simulink model "ssc_battery_rom_qbat"  (R2021a)
settings: Solver=ode1be  StartTime=0.0  StopTime=3600  FixedStep=elec_dt  RelTol=1e-3
PreLoadFcn:
  | % Model parameters
  | ssc_battery_rom_qbat_param
undefined symbols (not defined in the file or in its folder): coolant_flow_qoff, coolant_flow_Toff, coolant_flow_Ton, elec_dt, heat_dt, iniBatteryTemp, iniCoolantTemp, R0_mat, sigbuilder_block, SOC_vec, T_vec, V0_mat
libraries: fl_lib x47, nesl_utility x47, ee_lib x14
(part 3 of 3)

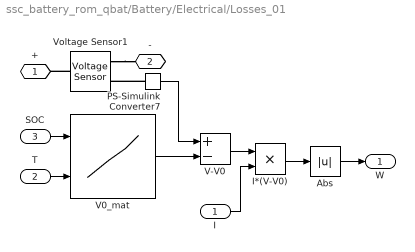
== system ssc_battery_rom_qbat/Battery/Electrical/Losses_01 ==
  I : Inport
  T : Inport  Port=2
  SOC : Inport  Port=3
  Abs : Abs
  I*(V-V0) : Product
  PS-Simulink Converter7 : nesl_utility/PS-Simulink Converter  PhysicalDomain=network_engine_domain  SubClassName=ps_output  LeftPortType=input  RightPortType=output  PseudoPeriodic=off  Frequencies=[]  Unit=inherit  AffineConversion=off
      settings: SourceProductBaseCode=PW,SS
  V-V0 : Sum  Inputs=+-
  V0_mat : Lookup_n-D  BreakpointsForDimension1=SOC_vec  BreakpointsForDimension2=T_vec  Table=V0_mat  InternalRulePriority=Speed  RndMeth=Simplest  InputSameDT=on
      settings: InputPortMap=u0,u1
  Voltage Sensor1 : fl_lib/Electrical/Electrical Sensors/Voltage Sensor
  + : PMIOPort  Side=Left
  - : PMIOPort  Port=2  Side=Right
  W : Outport
  wires:
  Abs/1 -> W/1
  PS-Simulink Converter7/1 -> V-V0/1
  I/1 -> I*(V-V0)/2
  I*(V-V0)/1 -> Abs/1
  V-V0/1 -> I*(V-V0)/1
  V0_mat/1 -> V-V0/2
  SOC/1 -> V0_mat/1
  T/1 -> V0_mat/2
  connections:
  PS-Simulink Converter7/LConn1 -- Voltage Sensor1/RConn1
  Voltage Sensor1/RConn2 -- -/RConn1
  Voltage Sensor1/LConn1 -- +/RConn1

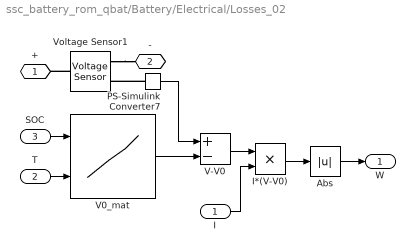
== system ssc_battery_rom_qbat/Battery/Electrical/Losses_02 ==
  I : Inport
  T : Inport  Port=2
  SOC : Inport  Port=3
  Abs : Abs
  I*(V-V0) : Product
  PS-Simulink Converter7 : nesl_utility/PS-Simulink Converter  PhysicalDomain=network_engine_domain  SubClassName=ps_output  LeftPortType=input  RightPortType=output  PseudoPeriodic=off  Frequencies=[]  Unit=inherit  AffineConversion=off
      settings: SourceProductBaseCode=PW,SS
  V-V0 : Sum  Inputs=+-
  V0_mat : Lookup_n-D  BreakpointsForDimension1=SOC_vec  BreakpointsForDimension2=T_vec  Table=V0_mat  InternalRulePriority=Speed  RndMeth=Simplest  InputSameDT=on
      settings: InputPortMap=u0,u1
  Voltage Sensor1 : fl_lib/Electrical/Electrical Sensors/Voltage Sensor
  + : PMIOPort  Side=Left
  - : PMIOPort  Port=2  Side=Right
  W : Outport
  wires:
  Abs/1 -> W/1
  PS-Simulink Converter7/1 -> V-V0/1
  I/1 -> I*(V-V0)/2
  I*(V-V0)/1 -> Abs/1
  V-V0/1 -> I*(V-V0)/1
  V0_mat/1 -> V-V0/2
  SOC/1 -> V0_mat/1
  T/1 -> V0_mat/2
  connections:
  PS-Simulink Converter7/LConn1 -- Voltage Sensor1/RConn1
  Voltage Sensor1/RConn2 -- -/RConn1
  Voltage Sensor1/LConn1 -- +/RConn1

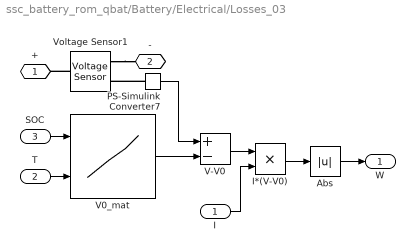
== system ssc_battery_rom_qbat/Battery/Electrical/Losses_03 ==
  I : Inport
  T : Inport  Port=2
  SOC : Inport  Port=3
  Abs : Abs
  I*(V-V0) : Product
  PS-Simulink Converter7 : nesl_utility/PS-Simulink Converter  PhysicalDomain=network_engine_domain  SubClassName=ps_output  LeftPortType=input  RightPortType=output  PseudoPeriodic=off  Frequencies=[]  Unit=inherit  AffineConversion=off
      settings: SourceProductBaseCode=PW,SS
  V-V0 : Sum  Inputs=+-
  V0_mat : Lookup_n-D  BreakpointsForDimension1=SOC_vec  BreakpointsForDimension2=T_vec  Table=V0_mat  InternalRulePriority=Speed  RndMeth=Simplest  InputSameDT=on
      settings: InputPortMap=u0,u1
  Voltage Sensor1 : fl_lib/Electrical/Electrical Sensors/Voltage Sensor
  + : PMIOPort  Side=Left
  - : PMIOPort  Port=2  Side=Right
  W : Outport
  wires:
  Abs/1 -> W/1
  PS-Simulink Converter7/1 -> V-V0/1
  I/1 -> I*(V-V0)/2
  I*(V-V0)/1 -> Abs/1
  V-V0/1 -> I*(V-V0)/1
  V0_mat/1 -> V-V0/2
  SOC/1 -> V0_mat/1
  T/1 -> V0_mat/2
  connections:
  PS-Simulink Converter7/LConn1 -- Voltage Sensor1/RConn1
  Voltage Sensor1/RConn2 -- -/RConn1
  Voltage Sensor1/LConn1 -- +/RConn1

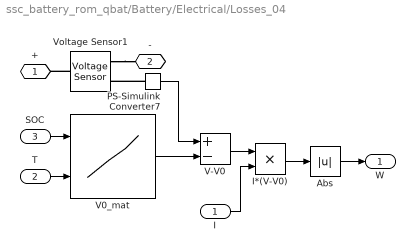
== system ssc_battery_rom_qbat/Battery/Electrical/Losses_04 ==
  I : Inport
  T : Inport  Port=2
  SOC : Inport  Port=3
  Abs : Abs
  I*(V-V0) : Product
  PS-Simulink Converter7 : nesl_utility/PS-Simulink Converter  PhysicalDomain=network_engine_domain  SubClassName=ps_output  LeftPortType=input  RightPortType=output  PseudoPeriodic=off  Frequencies=[]  Unit=inherit  AffineConversion=off
      settings: SourceProductBaseCode=PW,SS
  V-V0 : Sum  Inputs=+-
  V0_mat : Lookup_n-D  BreakpointsForDimension1=SOC_vec  BreakpointsForDimension2=T_vec  Table=V0_mat  InternalRulePriority=Speed  RndMeth=Simplest  InputSameDT=on
      settings: InputPortMap=u0,u1
  Voltage Sensor1 : fl_lib/Electrical/Electrical Sensors/Voltage Sensor
  + : PMIOPort  Side=Left
  - : PMIOPort  Port=2  Side=Right
  W : Outport
  wires:
  Abs/1 -> W/1
  PS-Simulink Converter7/1 -> V-V0/1
  I/1 -> I*(V-V0)/2
  I*(V-V0)/1 -> Abs/1
  V-V0/1 -> I*(V-V0)/1
  V0_mat/1 -> V-V0/2
  SOC/1 -> V0_mat/1
  T/1 -> V0_mat/2
  connections:
  PS-Simulink Converter7/LConn1 -- Voltage Sensor1/RConn1
  Voltage Sensor1/RConn2 -- -/RConn1
  Voltage Sensor1/LConn1 -- +/RConn1

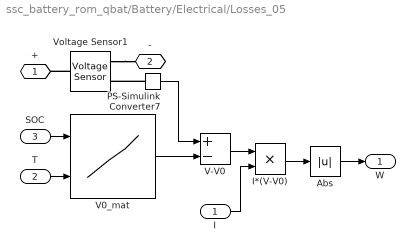
== system ssc_battery_rom_qbat/Battery/Electrical/Losses_05 ==
  I : Inport
  T : Inport  Port=2
  SOC : Inport  Port=3
  Abs : Abs
  I*(V-V0) : Product
  PS-Simulink Converter7 : nesl_utility/PS-Simulink Converter  PhysicalDomain=network_engine_domain  SubClassName=ps_output  LeftPortType=input  RightPortType=output  PseudoPeriodic=off  Frequencies=[]  Unit=inherit  AffineConversion=off
      settings: SourceProductBaseCode=PW,SS
  V-V0 : Sum  Inputs=+-
  V0_mat : Lookup_n-D  BreakpointsForDimension1=SOC_vec  BreakpointsForDimension2=T_vec  Table=V0_mat  InternalRulePriority=Speed  RndMeth=Simplest  InputSameDT=on
      settings: InputPortMap=u0,u1
  Voltage Sensor1 : fl_lib/Electrical/Electrical Sensors/Voltage Sensor
  + : PMIOPort  Side=Left
  - : PMIOPort  Port=2  Side=Right
  W : Outport
  wires:
  Abs/1 -> W/1
  PS-Simulink Converter7/1 -> V-V0/1
  I/1 -> I*(V-V0)/2
  I*(V-V0)/1 -> Abs/1
  V-V0/1 -> I*(V-V0)/1
  V0_mat/1 -> V-V0/2
  SOC/1 -> V0_mat/1
  T/1 -> V0_mat/2
  connections:
  PS-Simulink Converter7/LConn1 -- Voltage Sensor1/RConn1
  Voltage Sensor1/RConn2 -- -/RConn1
  Voltage Sensor1/LConn1 -- +/RConn1

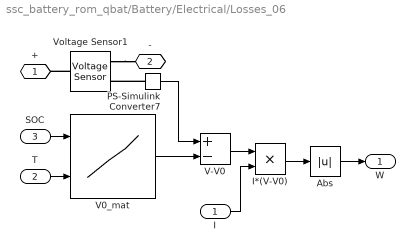
== system ssc_battery_rom_qbat/Battery/Electrical/Losses_06 ==
  I : Inport
  T : Inport  Port=2
  SOC : Inport  Port=3
  Abs : Abs
  I*(V-V0) : Product
  PS-Simulink Converter7 : nesl_utility/PS-Simulink Converter  PhysicalDomain=network_engine_domain  SubClassName=ps_output  LeftPortType=input  RightPortType=output  PseudoPeriodic=off  Frequencies=[]  Unit=inherit  AffineConversion=off
      settings: SourceProductBaseCode=PW,SS
  V-V0 : Sum  Inputs=+-
  V0_mat : Lookup_n-D  BreakpointsForDimension1=SOC_vec  BreakpointsForDimension2=T_vec  Table=V0_mat  InternalRulePriority=Speed  RndMeth=Simplest  InputSameDT=on
      settings: InputPortMap=u0,u1
  Voltage Sensor1 : fl_lib/Electrical/Electrical Sensors/Voltage Sensor
  + : PMIOPort  Side=Left
  - : PMIOPort  Port=2  Side=Right
  W : Outport
  wires:
  Abs/1 -> W/1
  PS-Simulink Converter7/1 -> V-V0/1
  I/1 -> I*(V-V0)/2
  I*(V-V0)/1 -> Abs/1
  V-V0/1 -> I*(V-V0)/1
  V0_mat/1 -> V-V0/2
  SOC/1 -> V0_mat/1
  T/1 -> V0_mat/2
  connections:
  PS-Simulink Converter7/LConn1 -- Voltage Sensor1/RConn1
  Voltage Sensor1/RConn2 -- -/RConn1
  Voltage Sensor1/LConn1 -- +/RConn1

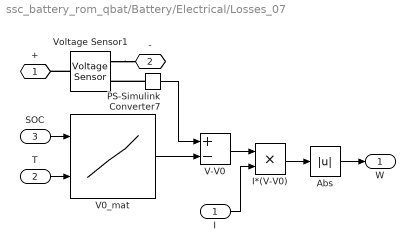
== system ssc_battery_rom_qbat/Battery/Electrical/Losses_07 ==
  I : Inport
  T : Inport  Port=2
  SOC : Inport  Port=3
  Abs : Abs
  I*(V-V0) : Product
  PS-Simulink Converter7 : nesl_utility/PS-Simulink Converter  PhysicalDomain=network_engine_domain  SubClassName=ps_output  LeftPortType=input  RightPortType=output  PseudoPeriodic=off  Frequencies=[]  Unit=inherit  AffineConversion=off
      settings: SourceProductBaseCode=PW,SS
  V-V0 : Sum  Inputs=+-
  V0_mat : Lookup_n-D  BreakpointsForDimension1=SOC_vec  BreakpointsForDimension2=T_vec  Table=V0_mat  InternalRulePriority=Speed  RndMeth=Simplest  InputSameDT=on
      settings: InputPortMap=u0,u1
  Voltage Sensor1 : fl_lib/Electrical/Electrical Sensors/Voltage Sensor
  + : PMIOPort  Side=Left
  - : PMIOPort  Port=2  Side=Right
  W : Outport
  wires:
  Abs/1 -> W/1
  PS-Simulink Converter7/1 -> V-V0/1
  I/1 -> I*(V-V0)/2
  I*(V-V0)/1 -> Abs/1
  V-V0/1 -> I*(V-V0)/1
  V0_mat/1 -> V-V0/2
  SOC/1 -> V0_mat/1
  T/1 -> V0_mat/2
  connections:
  PS-Simulink Converter7/LConn1 -- Voltage Sensor1/RConn1
  Voltage Sensor1/RConn2 -- -/RConn1
  Voltage Sensor1/LConn1 -- +/RConn1

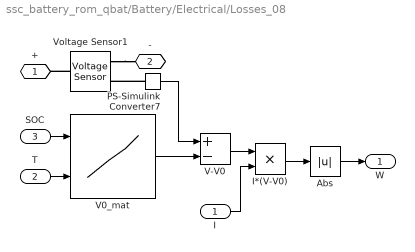
== system ssc_battery_rom_qbat/Battery/Electrical/Losses_08 ==
  I : Inport
  T : Inport  Port=2
  SOC : Inport  Port=3
  Abs : Abs
  I*(V-V0) : Product
  PS-Simulink Converter7 : nesl_utility/PS-Simulink Converter  PhysicalDomain=network_engine_domain  SubClassName=ps_output  LeftPortType=input  RightPortType=output  PseudoPeriodic=off  Frequencies=[]  Unit=inherit  AffineConversion=off
      settings: SourceProductBaseCode=PW,SS
  V-V0 : Sum  Inputs=+-
  V0_mat : Lookup_n-D  BreakpointsForDimension1=SOC_vec  BreakpointsForDimension2=T_vec  Table=V0_mat  InternalRulePriority=Speed  RndMeth=Simplest  InputSameDT=on
      settings: InputPortMap=u0,u1
  Voltage Sensor1 : fl_lib/Electrical/Electrical Sensors/Voltage Sensor
  + : PMIOPort  Side=Left
  - : PMIOPort  Port=2  Side=Right
  W : Outport
  wires:
  Abs/1 -> W/1
  PS-Simulink Converter7/1 -> V-V0/1
  I/1 -> I*(V-V0)/2
  I*(V-V0)/1 -> Abs/1
  V-V0/1 -> I*(V-V0)/1
  V0_mat/1 -> V-V0/2
  SOC/1 -> V0_mat/1
  T/1 -> V0_mat/2
  connections:
  PS-Simulink Converter7/LConn1 -- Voltage Sensor1/RConn1
  Voltage Sensor1/RConn2 -- -/RConn1
  Voltage Sensor1/LConn1 -- +/RConn1

== system ssc_battery_rom_qbat/Battery/Electrical/Losses_09 ==
  I : Inport
  T : Inport  Port=2
  SOC : Inport  Port=3
  Abs : Abs
  I*(V-V0) : Product
  PS-Simulink Converter7 : nesl_utility/PS-Simulink Converter  PhysicalDomain=network_engine_domain  SubClassName=ps_output  LeftPortType=input  RightPortType=output  PseudoPeriodic=off  Frequencies=[]  Unit=inherit  AffineConversion=off
      settings: SourceProductBaseCode=PW,SS
  V-V0 : Sum  Inputs=+-
  V0_mat : Lookup_n-D  BreakpointsForDimension1=SOC_vec  BreakpointsForDimension2=T_vec  Table=V0_mat  InternalRulePriority=Speed  RndMeth=Simplest  InputSameDT=on
      settings: InputPortMap=u0,u1
  Voltage Sensor1 : fl_lib/Electrical/Electrical Sensors/Voltage Sensor
  + : PMIOPort  Side=Left
  - : PMIOPort  Port=2  Side=Right
  W : Outport
  wires:
  Abs/1 -> W/1
  PS-Simulink Converter7/1 -> V-V0/1
  I/1 -> I*(V-V0)/2
  I*(V-V0)/1 -> Abs/1
  V-V0/1 -> I*(V-V0)/1
  V0_mat/1 -> V-V0/2
  SOC/1 -> V0_mat/1
  T/1 -> V0_mat/2
  connections:
  PS-Simulink Converter7/LConn1 -- Voltage Sensor1/RConn1
  Voltage Sensor1/RConn2 -- -/RConn1
  Voltage Sensor1/LConn1 -- +/RConn1

== system ssc_battery_rom_qbat/Battery/Electrical/Losses_10 ==
  I : Inport
  T : Inport  Port=2
  SOC : Inport  Port=3
  Abs : Abs
  I*(V-V0) : Product
  PS-Simulink Converter7 : nesl_utility/PS-Simulink Converter  PhysicalDomain=network_engine_domain  SubClassName=ps_output  LeftPortType=input  RightPortType=output  PseudoPeriodic=off  Frequencies=[]  Unit=inherit  AffineConversion=off
      settings: SourceProductBaseCode=PW,SS
  V-V0 : Sum  Inputs=+-
  V0_mat : Lookup_n-D  BreakpointsForDimension1=SOC_vec  BreakpointsForDimension2=T_vec  Table=V0_mat  InternalRulePriority=Speed  RndMeth=Simplest  InputSameDT=on
      settings: InputPortMap=u0,u1
  Voltage Sensor1 : fl_lib/Electrical/Electrical Sensors/Voltage Sensor
  + : PMIOPort  Side=Left
  - : PMIOPort  Port=2  Side=Right
  W : Outport
  wires:
  PS-Simulink Converter7/1 -> V-V0/1
  I/1 -> I*(V-V0)/2
  I*(V-V0)/1 -> Abs/1
  V-V0/1 -> I*(V-V0)/1
  V0_mat/1 -> V-V0/2
  SOC/1 -> V0_mat/1
  T/1 -> V0_mat/2
  Abs/1 -> W/1
  connections:
  PS-Simulink Converter7/LConn1 -- Voltage Sensor1/RConn1
  Voltage Sensor1/RConn2 -- -/RConn1
  Voltage Sensor1/LConn1 -- +/RConn1

== system ssc_battery_rom_qbat/Battery/Electrical/Losses_11 ==
  I : Inport
  T : Inport  Port=2
  SOC : Inport  Port=3
  Abs : Abs
  I*(V-V0) : Product
  PS-Simulink Converter7 : nesl_utility/PS-Simulink Converter  PhysicalDomain=network_engine_domain  SubClassName=ps_output  LeftPortType=input  RightPortType=output  PseudoPeriodic=off  Frequencies=[]  Unit=inherit  AffineConversion=off
      settings: SourceProductBaseCode=PW,SS
  V-V0 : Sum  Inputs=+-
  V0_mat : Lookup_n-D  BreakpointsForDimension1=SOC_vec  BreakpointsForDimension2=T_vec  Table=V0_mat  InternalRulePriority=Speed  RndMeth=Simplest  InputSameDT=on
      settings: InputPortMap=u0,u1
  Voltage Sensor1 : fl_lib/Electrical/Electrical Sensors/Voltage Sensor
  + : PMIOPort  Side=Left
  - : PMIOPort  Port=2  Side=Right
  W : Outport
  wires:
  Abs/1 -> W/1
  PS-Simulink Converter7/1 -> V-V0/1
  I/1 -> I*(V-V0)/2
  I*(V-V0)/1 -> Abs/1
  V-V0/1 -> I*(V-V0)/1
  V0_mat/1 -> V-V0/2
  SOC/1 -> V0_mat/1
  T/1 -> V0_mat/2
  connections:
  PS-Simulink Converter7/LConn1 -- Voltage Sensor1/RConn1
  Voltage Sensor1/RConn2 -- -/RConn1
  Voltage Sensor1/LConn1 -- +/RConn1

== system ssc_battery_rom_qbat/Battery/Electrical/Losses_12 ==
  I : Inport
  T : Inport  Port=2
  SOC : Inport  Port=3
  Abs : Abs
  I*(V-V0) : Product
  PS-Simulink Converter7 : nesl_utility/PS-Simulink Converter  PhysicalDomain=network_engine_domain  SubClassName=ps_output  LeftPortType=input  RightPortType=output  PseudoPeriodic=off  Frequencies=[]  Unit=inherit  AffineConversion=off
      settings: SourceProductBaseCode=PW,SS
  V-V0 : Sum  Inputs=+-
  V0_mat : Lookup_n-D  BreakpointsForDimension1=SOC_vec  BreakpointsForDimension2=T_vec  Table=V0_mat  InternalRulePriority=Speed  RndMeth=Simplest  InputSameDT=on
      settings: InputPortMap=u0,u1
  Voltage Sensor1 : fl_lib/Electrical/Electrical Sensors/Voltage Sensor
  + : PMIOPort  Side=Left
  - : PMIOPort  Port=2  Side=Right
  W : Outport
  wires:
  Abs/1 -> W/1
  PS-Simulink Converter7/1 -> V-V0/1
  I/1 -> I*(V-V0)/2
  I*(V-V0)/1 -> Abs/1
  V-V0/1 -> I*(V-V0)/1
  V0_mat/1 -> V-V0/2
  SOC/1 -> V0_mat/1
  T/1 -> V0_mat/2
  connections:
  PS-Simulink Converter7/LConn1 -- Voltage Sensor1/RConn1
  Voltage Sensor1/RConn2 -- -/RConn1
  Voltage Sensor1/LConn1 -- +/RConn1

== system ssc_battery_rom_qbat/Battery/Electrical/Losses_13 ==
  I : Inport
  T : Inport  Port=2
  SOC : Inport  Port=3
  Abs : Abs
  I*(V-V0) : Product
  PS-Simulink Converter7 : nesl_utility/PS-Simulink Converter  PhysicalDomain=network_engine_domain  SubClassName=ps_output  LeftPortType=input  RightPortType=output  PseudoPeriodic=off  Frequencies=[]  Unit=inherit  AffineConversion=off
      settings: SourceProductBaseCode=PW,SS
  V-V0 : Sum  Inputs=+-
  V0_mat : Lookup_n-D  BreakpointsForDimension1=SOC_vec  BreakpointsForDimension2=T_vec  Table=V0_mat  InternalRulePriority=Speed  RndMeth=Simplest  InputSameDT=on
      settings: InputPortMap=u0,u1
  Voltage Sensor1 : fl_lib/Electrical/Electrical Sensors/Voltage Sensor
  + : PMIOPort  Side=Left
  - : PMIOPort  Port=2  Side=Right
  W : Outport
  wires:
  Abs/1 -> W/1
  PS-Simulink Converter7/1 -> V-V0/1
  I/1 -> I*(V-V0)/2
  I*(V-V0)/1 -> Abs/1
  V-V0/1 -> I*(V-V0)/1
  V0_mat/1 -> V-V0/2
  SOC/1 -> V0_mat/1
  T/1 -> V0_mat/2
  connections:
  PS-Simulink Converter7/LConn1 -- Voltage Sensor1/RConn1
  Voltage Sensor1/RConn2 -- -/RConn1
  Voltage Sensor1/LConn1 -- +/RConn1

== system ssc_battery_rom_qbat/Battery/Electrical/Losses_14 ==
  I : Inport
  T : Inport  Port=2
  SOC : Inport  Port=3
  Abs : Abs
  I*(V-V0) : Product
  PS-Simulink Converter7 : nesl_utility/PS-Simulink Converter  PhysicalDomain=network_engine_domain  SubClassName=ps_output  LeftPortType=input  RightPortType=output  PseudoPeriodic=off  Frequencies=[]  Unit=inherit  AffineConversion=off
      settings: SourceProductBaseCode=PW,SS
  V-V0 : Sum  Inputs=+-
  V0_mat : Lookup_n-D  BreakpointsForDimension1=SOC_vec  BreakpointsForDimension2=T_vec  Table=V0_mat  InternalRulePriority=Speed  RndMeth=Simplest  InputSameDT=on
      settings: InputPortMap=u0,u1
  Voltage Sensor1 : fl_lib/Electrical/Electrical Sensors/Voltage Sensor
  + : PMIOPort  Side=Left
  - : PMIOPort  Port=2  Side=Right
  W : Outport
  wires:
  Abs/1 -> W/1
  PS-Simulink Converter7/1 -> V-V0/1
  I/1 -> I*(V-V0)/2
  I*(V-V0)/1 -> Abs/1
  V-V0/1 -> I*(V-V0)/1
  V0_mat/1 -> V-V0/2
  SOC/1 -> V0_mat/1
  T/1 -> V0_mat/2
  connections:
  PS-Simulink Converter7/LConn1 -- Voltage Sensor1/RConn1
  Voltage Sensor1/RConn2 -- -/RConn1
  Voltage Sensor1/LConn1 -- +/RConn1

== system ssc_battery_rom_qbat/Battery/Electrical/T_01 ==
  T : Inport
  273K : fl_lib/Thermal/Thermal Sources/Temperature Source  temperature=273 K
  Controlled Temperature Source : fl_lib/Thermal/Thermal Sources/Controlled Temperature Source
  Simulink-PS Converter1 : nesl_utility/Simulink-PS Converter  PhysicalDomain=network_engine_domain  SubClassName=ps_input  LeftPortType=input  RightPortType=output  PseudoPeriodic=off  Frequencies=[]  NoiseDistribution=none  NoiseParameters=[]  Unit=K  AffineConversion=off  FilteringAndDerivatives=filter  SimscapeFilterOrder=1  InputFilterTimeConstant=0.001  UdotUserProvided=0
      settings: SourceProductBaseCode=PW,SS
  B : PMIOPort  Side=Right
  wires:
  T/1 -> Simulink-PS Converter1/1
  connections:
  Simulink-PS Converter1/RConn1 -- Controlled Temperature Source/RConn1
  Controlled Temperature Source/LConn1 -- B/RConn1
  273K/LConn1 -- Controlled Temperature Source/RConn2

== system ssc_battery_rom_qbat/Battery/Electrical/T_02 ==
  T : Inport
  273K : fl_lib/Thermal/Thermal Sources/Temperature Source  temperature=273 K
  Controlled Temperature Source : fl_lib/Thermal/Thermal Sources/Controlled Temperature Source
  Simulink-PS Converter1 : nesl_utility/Simulink-PS Converter  PhysicalDomain=network_engine_domain  SubClassName=ps_input  LeftPortType=input  RightPortType=output  PseudoPeriodic=off  Frequencies=[]  NoiseDistribution=none  NoiseParameters=[]  Unit=K  AffineConversion=off  FilteringAndDerivatives=filter  SimscapeFilterOrder=1  InputFilterTimeConstant=0.001  UdotUserProvided=0
      settings: SourceProductBaseCode=PW,SS
  B : PMIOPort  Side=Right
  wires:
  T/1 -> Simulink-PS Converter1/1
  connections:
  Simulink-PS Converter1/RConn1 -- Controlled Temperature Source/RConn1
  Controlled Temperature Source/LConn1 -- B/RConn1
  273K/LConn1 -- Controlled Temperature Source/RConn2

== system ssc_battery_rom_qbat/Battery/Electrical/T_03 ==
  T : Inport
  273K : fl_lib/Thermal/Thermal Sources/Temperature Source  temperature=273 K
  Controlled Temperature Source : fl_lib/Thermal/Thermal Sources/Controlled Temperature Source
  Simulink-PS Converter1 : nesl_utility/Simulink-PS Converter  PhysicalDomain=network_engine_domain  SubClassName=ps_input  LeftPortType=input  RightPortType=output  PseudoPeriodic=off  Frequencies=[]  NoiseDistribution=none  NoiseParameters=[]  Unit=K  AffineConversion=off  FilteringAndDerivatives=filter  SimscapeFilterOrder=1  InputFilterTimeConstant=0.001  UdotUserProvided=0
      settings: SourceProductBaseCode=PW,SS
  B : PMIOPort  Side=Right
  wires:
  T/1 -> Simulink-PS Converter1/1
  connections:
  Simulink-PS Converter1/RConn1 -- Controlled Temperature Source/RConn1
  Controlled Temperature Source/LConn1 -- B/RConn1
  273K/LConn1 -- Controlled Temperature Source/RConn2

== system ssc_battery_rom_qbat/Battery/Electrical/T_04 ==
  T : Inport
  273K : fl_lib/Thermal/Thermal Sources/Temperature Source  temperature=273 K
  Controlled Temperature Source : fl_lib/Thermal/Thermal Sources/Controlled Temperature Source
  Simulink-PS Converter1 : nesl_utility/Simulink-PS Converter  PhysicalDomain=network_engine_domain  SubClassName=ps_input  LeftPortType=input  RightPortType=output  PseudoPeriodic=off  Frequencies=[]  NoiseDistribution=none  NoiseParameters=[]  Unit=K  AffineConversion=off  FilteringAndDerivatives=filter  SimscapeFilterOrder=1  InputFilterTimeConstant=0.001  UdotUserProvided=0
      settings: SourceProductBaseCode=PW,SS
  B : PMIOPort  Side=Right
  wires:
  T/1 -> Simulink-PS Converter1/1
  connections:
  Simulink-PS Converter1/RConn1 -- Controlled Temperature Source/RConn1
  Controlled Temperature Source/LConn1 -- B/RConn1
  273K/LConn1 -- Controlled Temperature Source/RConn2

== system ssc_battery_rom_qbat/Battery/Electrical/T_05 ==
  T : Inport
  273K : fl_lib/Thermal/Thermal Sources/Temperature Source  temperature=273 K
  Controlled Temperature Source : fl_lib/Thermal/Thermal Sources/Controlled Temperature Source
  Simulink-PS Converter1 : nesl_utility/Simulink-PS Converter  PhysicalDomain=network_engine_domain  SubClassName=ps_input  LeftPortType=input  RightPortType=output  PseudoPeriodic=off  Frequencies=[]  NoiseDistribution=none  NoiseParameters=[]  Unit=K  AffineConversion=off  FilteringAndDerivatives=filter  SimscapeFilterOrder=1  InputFilterTimeConstant=0.001  UdotUserProvided=0
      settings: SourceProductBaseCode=PW,SS
  B : PMIOPort  Side=Right
  wires:
  T/1 -> Simulink-PS Converter1/1
  connections:
  Simulink-PS Converter1/RConn1 -- Controlled Temperature Source/RConn1
  Controlled Temperature Source/LConn1 -- B/RConn1
  273K/LConn1 -- Controlled Temperature Source/RConn2

== system ssc_battery_rom_qbat/Battery/Electrical/T_06 ==
  T : Inport
  273K : fl_lib/Thermal/Thermal Sources/Temperature Source  temperature=273 K
  Controlled Temperature Source : fl_lib/Thermal/Thermal Sources/Controlled Temperature Source
  Simulink-PS Converter1 : nesl_utility/Simulink-PS Converter  PhysicalDomain=network_engine_domain  SubClassName=ps_input  LeftPortType=input  RightPortType=output  PseudoPeriodic=off  Frequencies=[]  NoiseDistribution=none  NoiseParameters=[]  Unit=K  AffineConversion=off  FilteringAndDerivatives=filter  SimscapeFilterOrder=1  InputFilterTimeConstant=0.001  UdotUserProvided=0
      settings: SourceProductBaseCode=PW,SS
  B : PMIOPort  Side=Right
  wires:
  T/1 -> Simulink-PS Converter1/1
  connections:
  Simulink-PS Converter1/RConn1 -- Controlled Temperature Source/RConn1
  Controlled Temperature Source/LConn1 -- B/RConn1
  273K/LConn1 -- Controlled Temperature Source/RConn2

== system ssc_battery_rom_qbat/Battery/Electrical/T_07 ==
  T : Inport
  273K : fl_lib/Thermal/Thermal Sources/Temperature Source  temperature=273 K
  Controlled Temperature Source : fl_lib/Thermal/Thermal Sources/Controlled Temperature Source
  Simulink-PS Converter1 : nesl_utility/Simulink-PS Converter  PhysicalDomain=network_engine_domain  SubClassName=ps_input  LeftPortType=input  RightPortType=output  PseudoPeriodic=off  Frequencies=[]  NoiseDistribution=none  NoiseParameters=[]  Unit=K  AffineConversion=off  FilteringAndDerivatives=filter  SimscapeFilterOrder=1  InputFilterTimeConstant=0.001  UdotUserProvided=0
      settings: SourceProductBaseCode=PW,SS
  B : PMIOPort  Side=Right
  wires:
  T/1 -> Simulink-PS Converter1/1
  connections:
  Simulink-PS Converter1/RConn1 -- Controlled Temperature Source/RConn1
  Controlled Temperature Source/LConn1 -- B/RConn1
  273K/LConn1 -- Controlled Temperature Source/RConn2

== system ssc_battery_rom_qbat/Battery/Electrical/T_08 ==
  T : Inport
  273K : fl_lib/Thermal/Thermal Sources/Temperature Source  temperature=273 K
  Controlled Temperature Source : fl_lib/Thermal/Thermal Sources/Controlled Temperature Source
  Simulink-PS Converter1 : nesl_utility/Simulink-PS Converter  PhysicalDomain=network_engine_domain  SubClassName=ps_input  LeftPortType=input  RightPortType=output  PseudoPeriodic=off  Frequencies=[]  NoiseDistribution=none  NoiseParameters=[]  Unit=K  AffineConversion=off  FilteringAndDerivatives=filter  SimscapeFilterOrder=1  InputFilterTimeConstant=0.001  UdotUserProvided=0
      settings: SourceProductBaseCode=PW,SS
  B : PMIOPort  Side=Right
  wires:
  T/1 -> Simulink-PS Converter1/1
  connections:
  Simulink-PS Converter1/RConn1 -- Controlled Temperature Source/RConn1
  Controlled Temperature Source/LConn1 -- B/RConn1
  273K/LConn1 -- Controlled Temperature Source/RConn2

== system ssc_battery_rom_qbat/Battery/Electrical/T_09 ==
  T : Inport
  273K : fl_lib/Thermal/Thermal Sources/Temperature Source  temperature=273 K
  Controlled Temperature Source : fl_lib/Thermal/Thermal Sources/Controlled Temperature Source
  Simulink-PS Converter1 : nesl_utility/Simulink-PS Converter  PhysicalDomain=network_engine_domain  SubClassName=ps_input  LeftPortType=input  RightPortType=output  PseudoPeriodic=off  Frequencies=[]  NoiseDistribution=none  NoiseParameters=[]  Unit=K  AffineConversion=off  FilteringAndDerivatives=filter  SimscapeFilterOrder=1  InputFilterTimeConstant=0.001  UdotUserProvided=0
      settings: SourceProductBaseCode=PW,SS
  B : PMIOPort  Side=Right
  wires:
  T/1 -> Simulink-PS Converter1/1
  connections:
  Simulink-PS Converter1/RConn1 -- Controlled Temperature Source/RConn1
  Controlled Temperature Source/LConn1 -- B/RConn1
  273K/LConn1 -- Controlled Temperature Source/RConn2

== system ssc_battery_rom_qbat/Battery/Electrical/T_10 ==
  T : Inport
  273K : fl_lib/Thermal/Thermal Sources/Temperature Source  temperature=273 K
  Controlled Temperature Source : fl_lib/Thermal/Thermal Sources/Controlled Temperature Source
  Simulink-PS Converter1 : nesl_utility/Simulink-PS Converter  PhysicalDomain=network_engine_domain  SubClassName=ps_input  LeftPortType=input  RightPortType=output  PseudoPeriodic=off  Frequencies=[]  NoiseDistribution=none  NoiseParameters=[]  Unit=K  AffineConversion=off  FilteringAndDerivatives=filter  SimscapeFilterOrder=1  InputFilterTimeConstant=0.001  UdotUserProvided=0
      settings: SourceProductBaseCode=PW,SS
  B : PMIOPort  Side=Right
  wires:
  T/1 -> Simulink-PS Converter1/1
  connections:
  Simulink-PS Converter1/RConn1 -- Controlled Temperature Source/RConn1
  Controlled Temperature Source/LConn1 -- B/RConn1
  273K/LConn1 -- Controlled Temperature Source/RConn2

== system ssc_battery_rom_qbat/Battery/Electrical/T_11 ==
  T : Inport
  273K : fl_lib/Thermal/Thermal Sources/Temperature Source  temperature=273 K
  Controlled Temperature Source : fl_lib/Thermal/Thermal Sources/Controlled Temperature Source
  Simulink-PS Converter1 : nesl_utility/Simulink-PS Converter  PhysicalDomain=network_engine_domain  SubClassName=ps_input  LeftPortType=input  RightPortType=output  PseudoPeriodic=off  Frequencies=[]  NoiseDistribution=none  NoiseParameters=[]  Unit=K  AffineConversion=off  FilteringAndDerivatives=filter  SimscapeFilterOrder=1  InputFilterTimeConstant=0.001  UdotUserProvided=0
      settings: SourceProductBaseCode=PW,SS
  B : PMIOPort  Side=Right
  wires:
  T/1 -> Simulink-PS Converter1/1
  connections:
  Simulink-PS Converter1/RConn1 -- Controlled Temperature Source/RConn1
  Controlled Temperature Source/LConn1 -- B/RConn1
  273K/LConn1 -- Controlled Temperature Source/RConn2

== system ssc_battery_rom_qbat/Battery/Electrical/T_12 ==
  T : Inport
  273K : fl_lib/Thermal/Thermal Sources/Temperature Source  temperature=273 K
  Controlled Temperature Source : fl_lib/Thermal/Thermal Sources/Controlled Temperature Source
  Simulink-PS Converter1 : nesl_utility/Simulink-PS Converter  PhysicalDomain=network_engine_domain  SubClassName=ps_input  LeftPortType=input  RightPortType=output  PseudoPeriodic=off  Frequencies=[]  NoiseDistribution=none  NoiseParameters=[]  Unit=K  AffineConversion=off  FilteringAndDerivatives=filter  SimscapeFilterOrder=1  InputFilterTimeConstant=0.001  UdotUserProvided=0
      settings: SourceProductBaseCode=PW,SS
  B : PMIOPort  Side=Right
  wires:
  T/1 -> Simulink-PS Converter1/1
  connections:
  Simulink-PS Converter1/RConn1 -- Controlled Temperature Source/RConn1
  Controlled Temperature Source/LConn1 -- B/RConn1
  273K/LConn1 -- Controlled Temperature Source/RConn2

== system ssc_battery_rom_qbat/Battery/Electrical/T_13 ==
  T : Inport
  273K : fl_lib/Thermal/Thermal Sources/Temperature Source  temperature=273 K
  Controlled Temperature Source : fl_lib/Thermal/Thermal Sources/Controlled Temperature Source
  Simulink-PS Converter1 : nesl_utility/Simulink-PS Converter  PhysicalDomain=network_engine_domain  SubClassName=ps_input  LeftPortType=input  RightPortType=output  PseudoPeriodic=off  Frequencies=[]  NoiseDistribution=none  NoiseParameters=[]  Unit=K  AffineConversion=off  FilteringAndDerivatives=filter  SimscapeFilterOrder=1  InputFilterTimeConstant=0.001  UdotUserProvided=0
      settings: SourceProductBaseCode=PW,SS
  B : PMIOPort  Side=Right
  wires:
  T/1 -> Simulink-PS Converter1/1
  connections:
  Simulink-PS Converter1/RConn1 -- Controlled Temperature Source/RConn1
  Controlled Temperature Source/LConn1 -- B/RConn1
  273K/LConn1 -- Controlled Temperature Source/RConn2

== system ssc_battery_rom_qbat/Battery/Electrical/T_14 ==
  T : Inport
  273K : fl_lib/Thermal/Thermal Sources/Temperature Source  temperature=273 K
  Controlled Temperature Source : fl_lib/Thermal/Thermal Sources/Controlled Temperature Source
  Simulink-PS Converter1 : nesl_utility/Simulink-PS Converter  PhysicalDomain=network_engine_domain  SubClassName=ps_input  LeftPortType=input  RightPortType=output  PseudoPeriodic=off  Frequencies=[]  NoiseDistribution=none  NoiseParameters=[]  Unit=K  AffineConversion=off  FilteringAndDerivatives=filter  SimscapeFilterOrder=1  InputFilterTimeConstant=0.001  UdotUserProvided=0
      settings: SourceProductBaseCode=PW,SS
  B : PMIOPort  Side=Right
  wires:
  T/1 -> Simulink-PS Converter1/1
  connections:
  Simulink-PS Converter1/RConn1 -- Controlled Temperature Source/RConn1
  Controlled Temperature Source/LConn1 -- B/RConn1
  273K/LConn1 -- Controlled Temperature Source/RConn2

== system ssc_battery_rom_qbat/Battery/Electrical/Voltage Sensor ==
  PS-Simulink Converter : nesl_utility/PS-Simulink Converter  PhysicalDomain=network_engine_domain  SubClassName=ps_output  LeftPortType=input  RightPortType=output  PseudoPeriodic=off  Frequencies=[]  Unit=V  AffineConversion=off
      settings: SourceProductBaseCode=PW,SS
  Voltage Sensor : fl_lib/Electrical/Electrical Sensors/Voltage Sensor
  + : PMIOPort  Side=Left
  - : PMIOPort  Port=2  Side=Right
  voltage : Outport
  wires:
  PS-Simulink Converter/1 -> voltage/1
  connections:
  Voltage Sensor/RConn1 -- PS-Simulink Converter/LConn1
  +/RConn1 -- Voltage Sensor/LConn1
  -/RConn1 -- Voltage Sensor/RConn2
